simulink model "Model_controlled"  (Simulink 8.3)
settings: Solver=ode45  StartTime=tstart  StopTime=2000  RelTol=1e-3
values from neighbouring files (symbols this model uses):
  K = 3.54    [task1.m]
  T = 117.52    [task1.m]
undefined symbols (not defined in the file or in its folder): c_ss
libraries: simulink_extras x1
settings Model: Creator=christh  LastModifiedBy=Hwk  ExtModeAutoUpdateStatusClock=off
settings OptimizationCC: ExpressionDepthLimit=2147483647  InitFltsAndDblsToZero=on
settings DebuggingCC: FcnCallInpInsideContextMsg=UseLocalSettings

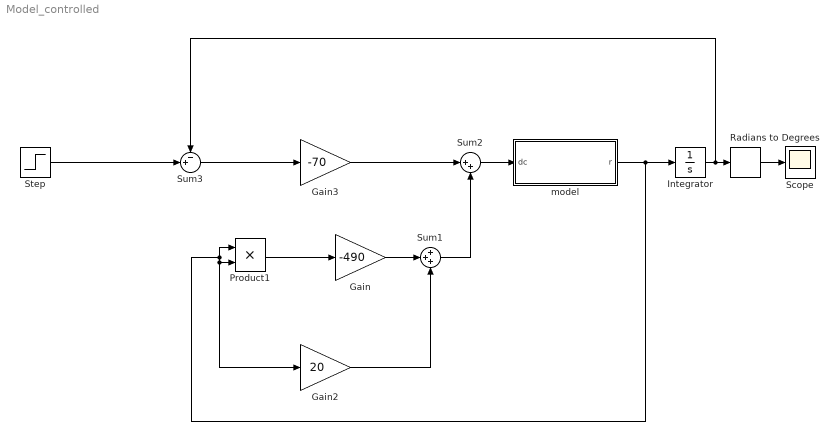
== system Model_controlled ==
  Gain : Gain  Gain=-490
  Gain2 : Gain  Gain=20
  Gain3 : Gain  Gain=-70
  Integrator : Integrator
  Product1 : Product
  Radians to Degrees : simulink_extras/Transformations/Radians to Degrees
  Scope : Scope
      settings: TimeRange=700  YMin=-32500  YMax=-28500
  Step : Step  Time=0  After=deg2rad(18)  SampleTime=0
  Sum1 : Sum  Inputs=+++
  Sum2 : Sum  Inputs=|++
  Sum3 : Sum  Inputs=-+|
  model : Subsystem
  wires:
  model/1(r) -> Product1/1, Gain2/1, Product1/2, Integrator/1
  Product1/1 -> Gain/1
  Integrator/1 -> Sum3/1, Radians to Degrees/1
  Gain2/1 -> Sum1/3
  Gain/1 -> Sum1/2
  Radians to Degrees/1 -> Scope/1
  Sum1/1 -> Sum2/2
  Sum2/1 -> model/1(dc)
  Step/1 -> Sum3/2
  Sum3/1 -> Gain3/1
  Gain3/1 -> Sum2/1

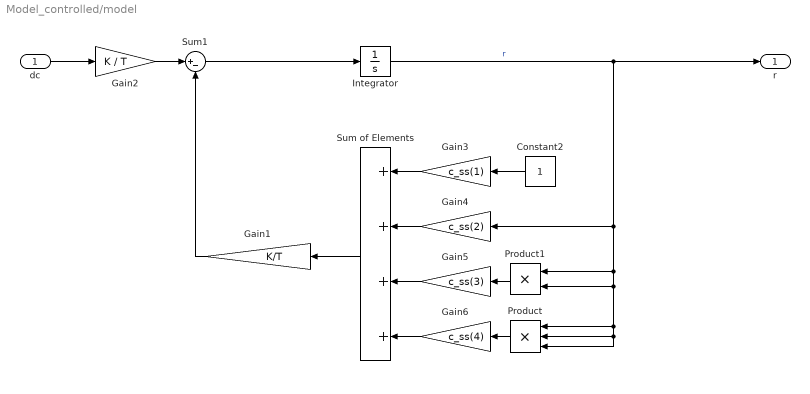
== system Model_controlled/model ==
  dc : Inport
  Constant2 : Constant
  Gain1 : Gain  Gain=K/T
  Gain2 : Gain  Gain=K / T
  Gain3 : Gain  Gain=c_ss(1)
  Gain4 : Gain  Gain=c_ss(2)
  Gain5 : Gain  Gain=c_ss(3)
  Gain6 : Gain  Gain=c_ss(4)
  Integrator : Integrator
  Product : Product  Inputs=3
  Product1 : Product
  Sum of Elements : Sum  Inputs=4
  Sum1 : Sum  Inputs=|+-
  r : Outport
  wires:
  Sum1/1 -> Integrator/1
  Gain1/1 -> Sum1/2
  dc/1 -> Gain2/1
  Gain2/1 -> Sum1/1
  Sum of Elements/1 -> Gain1/1
  Gain4/1 -> Sum of Elements/2
  Gain5/1 -> Sum of Elements/3
  Gain6/1 -> Sum of Elements/4
  Gain3/1 -> Sum of Elements/1
  Integrator/1 -> r/1, Gain4/1, Product/3, Product/2, Product/1, Product1/2, Product1/1  "r"
  Constant2/1 -> Gain3/1
  Product1/1 -> Gain5/1
  Product/1 -> Gain6/1
